simulink model "generic_20240709_1553"  (R2022a)
settings: Solver=ode45  StartTime=0.0  StopTime=inf  RelTol=1e-3  EnableMultiTasking=on
libraries: CarMaker4SL x40, simulink x9, aerolibconvert2 x4, matrix_library x4
(part 1 of 2)
settings Model: Creator=fh  LastModifiedBy=TFTS06
settings SolverCC: AlgebraicLoopSolver=TrustRegion
settings DataIOCC: LimitDataPoints=on  SaveFormat=Array  SignalLoggingSaveFormat=ModelDataLogs  ReturnWorkspaceOutputs=off  SignalLoggingName=sigsOut
settings OptimizationCC: BooleanDataType=off  ExpressionDepthLimit=2147483647  InitFltsAndDblsToZero=on  LifeSpan=inf
settings DebuggingCC: SaveWithParameterizedLinksMsg=none  UnderspecifiedInitializationDetection=Classic  MergeDetectMultiDrivingBlocksExec=none  SignalResolutionControl=TryResolveAllWithWarning  MultiTaskDSMMsg=warning  MultiTaskCondExecSysMsg=none  FcnCallInpInsideContextMsg=warning  UnconnectedInputMsg=warning  UnconnectedOutputMsg=warning  UnconnectedLineMsg=warning  StateNameClashWarn=warning  SFUnexpectedBacktrackingDiag=warning  SFNoUnconditionalDefaultTransitionDiag=warning  SFMachineParentedDataDiag=warning  ArithmeticOperatorsInVariantConditions=warning
settings HardwareCC: ProdBitPerPointer=32  ProdBitPerSizeT=32  ProdBitPerPtrDiffT=32  ProdLargestAtomicFloat=None  ProdIntDivRoundTo=Undefined  ProdEndianess=Unspecified  ProdWordSize=32  ProdHWDeviceType=32-bit Generic  TargetUnknown=on
settings ModelReferenceCC: PropagateSignalLabelsOutOfModel=off
settings SFSimCC: SimUseLocalCustomCode=off  CustomCodeUndefinedFunction=UseInterfaceOnly
settings RTWCC: RTWUseLocalCustomCode=off
settings CodeAppCC: MaxIdLength=63  StateflowObjectComments=on
settings GRTTargetCC: TargetFcnLib=ansi_tfl_tmw.mat  TargetLangStandard=C89/C90 (ANSI)  CombineOutputUpdateFcns=off  GRTInterface=on
settings ConfigComp: CovMetricSettings=dw  CovSaveCumulativeToWorkspaceVar=on  CovSaveSingleToWorkspaceVar=on  CovExternalEMLEnable=off

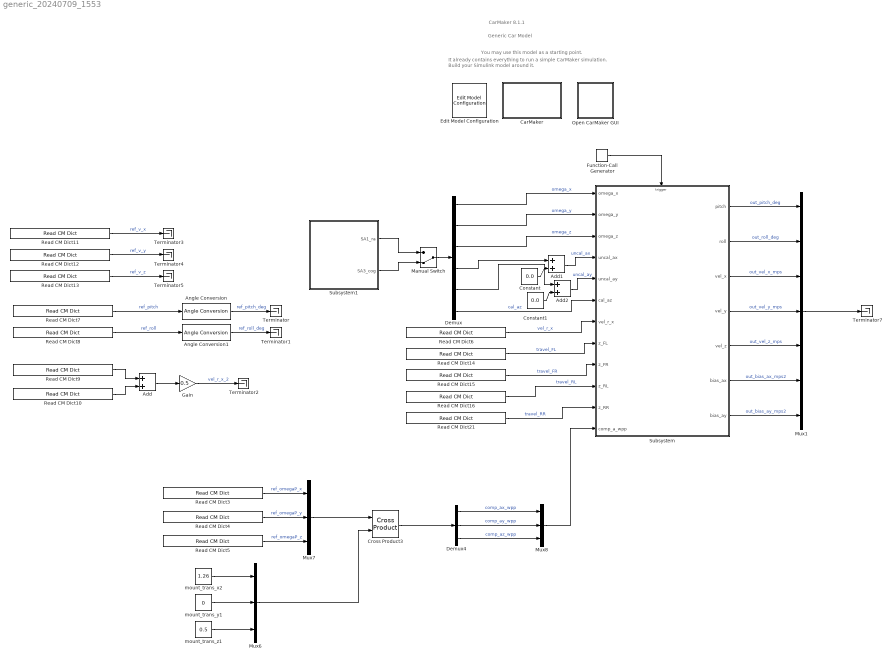
== system generic_20240709_1553 ==
  note: Generic Car Model
  note: You may use this model as a starting point.
  note: It already contains everything to run a simple CarMaker simulation.
      | Build your Simulink model around it.
  note: CarMaker 8.1.1
  Add : Sum
  Add1 : Sum
  Add2 : Sum
  Angle Conversion : aerolibconvert2/Angle Conversion  IU=rad  OU=deg
  Angle Conversion1 : aerolibconvert2/Angle Conversion  IU=rad  OU=deg
  CarMaker : Subsystem  TreatAsAtomicUnit=on
      mask Display: image(imread('CarMakerSys.png'));
  Constant : Constant  Value=0.0
  Constant1 : Constant  Value=0.0
  Cross Product3 : matrix_library/Cross Product
      settings: SourceProductBaseCode=SL
  Demux : Demux  Outputs=6
  Demux4 : Demux  Outputs=3
  Edit Model Configuration : CarMaker4SL/Edit Model Configuration  SFunctionModules=''
  Function-Call Generator : simulink/Ports & Subsystems/Function-Call Generator  sample_time=0.01  numberOfIterations=1  DisallowWideOutput=off
  Gain : Gain  Gain=0.5
  Manual Switch : ManualSwitch  CurrentSetting=0
  Mux1 : Mux  Inputs=7
  Mux6 : Mux  Inputs=3
  Mux7 : Mux  Inputs=3
  Mux8 : Mux  Inputs=3
  Open CarMaker GUI : Subsystem  LoadFcn=if ~length(which('cmself')), cmenv; end
      settings: OpenFcn=cmblockmagic('gui_fix_display'); CM_Simulink
      mask Display: image(imread('CarMakerGUI.png'));
  Read CM Dict10 : CarMaker4SL/Read CM Dict  xname=Car.vRR  xsync=off
  Read CM Dict11 : CarMaker4SL/Read CM Dict  xname=Sensor.Inertial.SA1.Vel_B.x  xsync=off
  Read CM Dict12 : CarMaker4SL/Read CM Dict  xname=Sensor.Inertial.SA1.Vel_B.y  xsync=off
  Read CM Dict13 : CarMaker4SL/Read CM Dict  xname=Sensor.Inertial.SA1.Vel_B.z  xsync=off
  Read CM Dict14 : CarMaker4SL/Read CM Dict  xname=Car.DampFL.l_kin  xsync=off
  Read CM Dict15 : CarMaker4SL/Read CM Dict  xname=Car.DampFR.l_kin  xsync=off
  Read CM Dict16 : CarMaker4SL/Read CM Dict  xname=Car.DampRL.l_kin  xsync=off
  Read CM Dict21 : CarMaker4SL/Read CM Dict  xname=Car.DampRR.l_kin  xsync=off
  Read CM Dict3 : CarMaker4SL/Read CM Dict  xname=Sensor.Inertial.SA1.Alpha_B.x  xsync=off
  Read CM Dict4 : CarMaker4SL/Read CM Dict  xname=Sensor.Inertial.SA1.Alpha_B.y  xsync=off
  Read CM Dict5 : CarMaker4SL/Read CM Dict  xname=Sensor.Inertial.SA1.Alpha_B.z  xsync=off
  Read CM Dict6 : CarMaker4SL/Read CM Dict  xname=Car.vx  xsync=off
  Read CM Dict7 : CarMaker4SL/Read CM Dict  xname=Car.Pitch  xsync=off
  Read CM Dict8 : CarMaker4SL/Read CM Dict  xname=Car.Roll  xsync=off
  Read CM Dict9 : CarMaker4SL/Read CM Dict  xname=Car.vRL  xsync=off
  Subsystem : Subsystem
  Subsystem1 : Subsystem
  Terminator{,1..5,7} (7 alike) : Terminator
  mount_trans_x2 : Constant  Value=1.26
  mount_trans_y1 : Constant  Value=0
  mount_trans_z1 : Constant  Value=0.5
  wires:
  Add1/1 -> Subsystem/4(uncal_ax)  "uncal_ax"
  Add2/1 -> Subsystem/5(uncal_ay)  "uncal_ay"
  Read CM Dict6/1 -> Subsystem/7(vel_r_x)  "vel_r_x"
  Read CM Dict7/1 -> Angle Conversion/1  "ref_pitch"
  Read CM Dict8/1 -> Angle Conversion1/1  "ref_roll"
  Subsystem/1(pitch) -> Mux1/1  "out_pitch_deg"
  Subsystem/7(bias_ay) -> Mux1/7  "out_bias_ay_mps2"
  Subsystem/6(bias_ax) -> Mux1/6  "out_bias_ax_mps2"
  Subsystem/4(vel_y) -> Mux1/4  "out_vel_y_mps"
  Subsystem/3(vel_x) -> Mux1/3  "out_vel_x_mps"
  Mux1/1 -> Terminator7/1
  Subsystem/5(vel_z) -> Mux1/5  "out_vel_z_mps"
  Subsystem/2(roll) -> Mux1/2  "out_roll_deg"
  Function-Call Generator/1 -> Subsystem/Trigger
  Angle Conversion/1 -> Terminator/1  "ref_pitch_deg"
  Angle Conversion1/1 -> Terminator1/1  "ref_roll_deg"
  Read CM Dict9/1 -> Add/1
  Read CM Dict10/1 -> Add/2
  Add/1 -> Gain/1
  Gain/1 -> Terminator2/1  "vel_r_x_2"
  Read CM Dict11/1 -> Terminator3/1  "ref_v_x"
  Read CM Dict13/1 -> Terminator5/1  "ref_v_z"
  Read CM Dict12/1 -> Terminator4/1  "ref_v_y"
  Constant/1 -> Add1/2
  Read CM Dict14/1 -> Subsystem/8(z_FL)  "travel_FL"
  Read CM Dict15/1 -> Subsystem/9(z_FR)  "travel_FR"
  Read CM Dict16/1 -> Subsystem/10(z_RL)  "travel_RL"
  Read CM Dict21/1 -> Subsystem/11(z_RR)  "travel_RR"
  Constant1/1 -> Add2/2
  Demux/1 -> Subsystem/1(omega_x)  "omega_x"
  Demux/2 -> Subsystem/2(omega_y)  "omega_y"
  Demux/3 -> Subsystem/3(omega_z)  "omega_z"
  Demux/4 -> Add1/1
  Demux/5 -> Add2/1
  Demux/6 -> Subsystem/6(cal_az)  "cal_az"
  Manual Switch/1 -> Demux/1
  Subsystem1/1(SA1_ra) -> Manual Switch/1
  Subsystem1/2(SA3_cog) -> Manual Switch/2
  Cross Product3/1 -> Demux4/1
  Read CM Dict5/1 -> Mux7/3  "ref_omegaP_z"
  Read CM Dict3/1 -> Mux7/1  "ref_omegaP_x"
  Mux8/1 -> Subsystem/12(comp_a_wpp)
  Mux7/1 -> Cross Product3/1
  mount_trans_z1/1 -> Mux6/3
  mount_trans_y1/1 -> Mux6/2
  Read CM Dict4/1 -> Mux7/2  "ref_omegaP_y"
  Demux4/3 -> Mux8/3  "comp_az_wpp"
  Demux4/2 -> Mux8/2  "comp_ay_wpp"
  Mux6/1 -> Cross Product3/2
  mount_trans_x2/1 -> Mux6/1
  Demux4/1 -> Mux8/1  "comp_ax_wpp"

== system generic_20240709_1553/CarMaker ==
  CM_FIRST : Subsystem
  CM_LAST : Subsystem
  DrivMan : Subsystem
  Ground : Ground
  IPG Vehicle : Subsystem  TreatAsAtomicUnit=on
  Terminator : Terminator
  VehicleControl : Subsystem
  wires:
  DrivMan/2(DrivMan.Out) -> VehicleControl/2(DrivMan.In)
  DrivMan/1(Sync_Out) -> VehicleControl/1(Sync_In)
  CM_FIRST/2(Env.Misc) -> DrivMan/2(Env.Misc)
  CM_FIRST/1(Sync_Out) -> DrivMan/1(Sync_In)
  CM_LAST/1(Sync_Out) -> Terminator/1
  Ground/1 -> CM_FIRST/1(Sync_In)
  IPG Vehicle/1(Sync_Out) -> CM_LAST/1(Sync_In)
  VehicleControl/1(Sync_Out) -> IPG Vehicle/1(Sync_In)
  VehicleControl/3(VhclCtrl.Steering) -> IPG Vehicle/3(VhclCtrl.Steering)
  VehicleControl/4(Vhcl.Wheel.In) -> IPG Vehicle/4(Vhcl.Wheel.In)
  VehicleControl/5(Vhcl.Misc) -> IPG Vehicle/5(Vhcl.Misc)
  VehicleControl/6(VhclCtrl.Brake) -> IPG Vehicle/6(VhclCtrl.Brake)
  VehicleControl/7(VhclCtrl.PT) -> IPG Vehicle/7(VhclCtrl.PT)
  VehicleControl/2(Vhcl.Model.Source) -> IPG Vehicle/2(Vhcl.Model.Source)

== system generic_20240709_1553/Open CarMaker GUI ==
  S-Function : S-Function  FunctionName=cm_gui  SFunctionDeploymentMode=off  EnableBusSupport=off

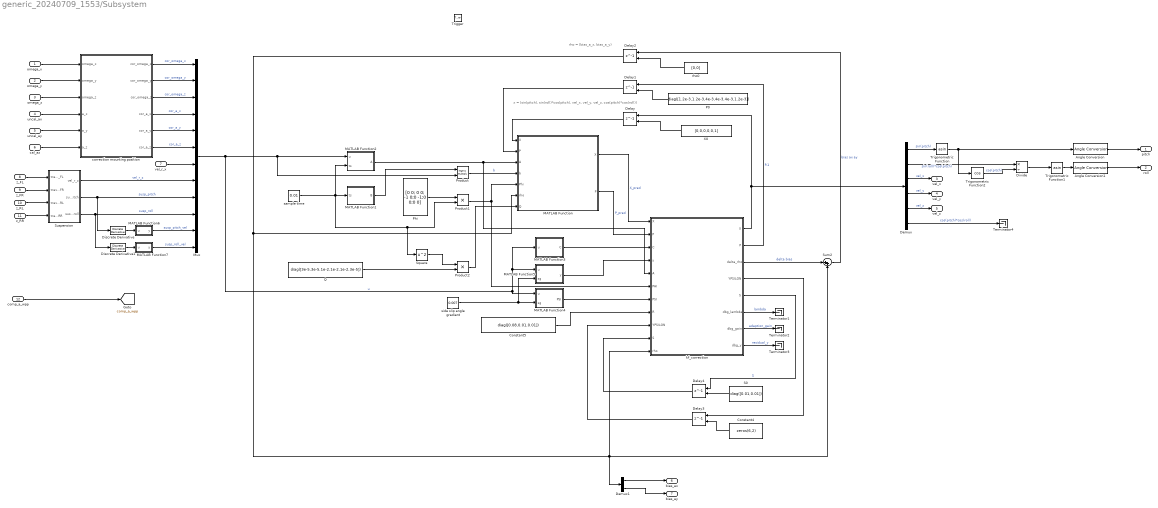
== system generic_20240709_1553/Subsystem ==
  note: rho = (bias_a_x, bias_a_y)
  note: x = (sin(pitch), sin(roll)*cos(pitch), vel_x, vel_y, vel_z, cos(pitch)*cos(roll))
  omega_x : Inport
  omega_y : Inport  Port=2
  omega_z : Inport  Port=3
  uncal_ax : Inport  Port=4
  uncal_ay : Inport  Port=5
  cal_az : Inport  Port=6
  vel_r_x : Inport  Port=7
  z_FL : Inport  Port=8
  z_FR : Inport  Port=9
  z_RL : Inport  Port=10
  z_RR : Inport  Port=11
  comp_a_wpp : Inport  Port=12
  Trigger : TriggerPort  TriggerType=function-call  VariantControl=(inherit)  PortDimensions=1
  Angle Conversion : aerolibconvert2/Angle Conversion  IU=rad  OU=deg
  Angle Conversion1 : aerolibconvert2/Angle Conversion  IU=rad  OU=deg
  Constant4 : Constant  Value=zeros(6,2)
  Constant5 : Constant  Value=diag([0.08,0.01,0.01])
  Delay{,1..4} (5 alike) : Delay  DelayLength=1  InitialConditionSource=Input port  InitialCondition=0
      settings: InputPortMap=u0,p4
  Demux : Demux  Outputs=6
  Demux1 : Demux  Outputs=2
  Discrete Derivative : simulink/Discrete/Discrete Derivative  gainval=1.0  ICPrevScaledInput=0.0  OutMin=[]  OutMax=[]  OutDataType=fixdt(1, 16)  OutScaling=2^-10  DoSatur=off
  Discrete Derivative1 : simulink/Discrete/Discrete Derivative  gainval=1.0  ICPrevScaledInput=0.0  OutMin=[]  OutMax=[]  OutDataType=fixdt(1, 16)  OutScaling=2^-10  DoSatur=off
  Divide : Product  Inputs=*/
  MATLAB Function : MATLAB Function  TreatAsAtomicUnit=on
  MATLAB Function1 : MATLAB Function  TreatAsAtomicUnit=on
  MATLAB Function2 : MATLAB Function  TreatAsAtomicUnit=on
  MATLAB Function3 : MATLAB Function  TreatAsAtomicUnit=on
  MATLAB Function4 : MATLAB Function  TreatAsAtomicUnit=on
  MATLAB Function5 : MATLAB Function  TreatAsAtomicUnit=on
  MATLAB Function6 : MATLAB Function  TreatAsAtomicUnit=on
  MATLAB Function7 : MATLAB Function  TreatAsAtomicUnit=on
  Mux : Mux  Inputs=12
  P0 : Constant  Value=diag([1.2e-3,1.2e-3,4e-3,4e-3,4e-3,1.2e-3])
  Phi : Constant  Value=[0 0; 0 0; -1 0;0 -1;0 0;0 0]
  Product : Product  Multiplication=Matrix(*)
  Product1 : Product
  Product2 : Product
  Q : Constant  Value=diag([3e-5,3e-5,1e-2,1e-2,1e-2,3e-5])
  S0 : Constant  Value=diag([0.01,0.01])
  Square : Math  Operator=square
  Sum2 : Sum  Inputs=|++
  Suspension : Subsystem
  Terminator{1..4} (4 alike) : Terminator
  Trigonometric Function : Trigonometry  Operator=asin
  Trigonometric Function1 : Trigonometry  Operator=asin
  Trigonometric Function2 : Trigonometry  Operator=cos
  X0 : Constant  Value=[0,0,0,0,0,1]
  correction mounting position : Subsystem
  kf_correction : MATLAB Function  TreatAsAtomicUnit=on
  rho0 : Constant  Value=[0,0]
  sample time : Constant  Value=0.01
  side slip angle gradient : Constant  Value=0.007
  pitch : Outport
  roll : Outport  Port=2
  vel_x : Outport  Port=3
  vel_y : Outport  Port=4
  vel_z : Outport  Port=5
  bias_ax : Outport  Port=6
  bias_ay : Outport  Port=7
  tag scope: comp_a_wpp=global
  wires:
  Demux1/2 -> bias_ay/1
  kf_correction/5(S) -> Delay4/1  "S"
  X0/1 -> Delay/2
  kf_correction/7(dbg_gain) -> Terminator2/1  "adaption_gain"
  Demux/1 -> Trigonometric Function/1  "sin(pitch)"
  P0/1 -> Delay1/2
  Demux/3 -> vel_x/1  "vel_x"
  Product/1 -> MATLAB Function/4(b)  "b"
  kf_correction/1(X) -> Demux/1, Delay/1
  Constant4/1 -> Delay3/2
  Demux/4 -> vel_y/1  "vel_y"
  Divide/1 -> Trigonometric Function1/1
  MATLAB Function2/1(A) -> kf_correction/5(A), MATLAB Function/3(A)
  Phi/1 -> Product1/1
  Demux1/1 -> bias_ax/1
  Delay/1 -> MATLAB Function/1("X ")
  MATLAB Function3/1(C) -> kf_correction/3(C)
  kf_correction/2(P) -> Delay1/1  "P-1"
  Suspension/2(susp_pitch) -> Mux/9, Discrete Derivative/1  "susp_pitch"
  Demux/2 -> Divide/1  "sin(roll)*cos(pitch)"
  Delay4/1 -> kf_correction/10("S ")
  Mux/1 -> MATLAB Function2/1(u), Product/2, MATLAB Function4/1(u), MATLAB Function3/1(u), MATLAB Function5/1(u)  "u"
  Suspension/3(susp_roll) -> Mux/10, Discrete Derivative1/1  "susp_roll"
  kf_correction/3(delta_rho) -> Sum2/1  "delta bias"
  Sum2/1 -> Delay2/1  "bias ax ay"
  Trigonometric Function/1 -> Angle Conversion/1, Trigonometric Function2/1
  Constant5/1 -> kf_correction/8(R)
  MATLAB Function4/1(PSI) -> kf_correction/7(PSI)
  Delay3/1 -> kf_correction/9("YPSILON ")
  Suspension/1(vel_r_z) -> Mux/8  "vel_r_z"
  S0/1 -> Delay4/2
  MATLAB Function1/1(B) -> Product/1
  Delay1/1 -> MATLAB Function/2("P ")
  Product1/1 -> MATLAB Function/5(Phi), kf_correction/6(PHI)
  MATLAB Function/2(P) -> kf_correction/2("P ")  "P_pred"
  Trigonometric Function1/1 -> Angle Conversion1/1
  Demux/5 -> vel_z/1  "vel_z"
  rho0/1 -> Delay2/2
  sample time/1 -> MATLAB Function2/2(ts), Product1/2, Square/1, MATLAB Function1/1(ts)
  MATLAB Function/1(X) -> kf_correction/1("X ")  "X_pred"
  Trigonometric Function2/1 -> Divide/2  "cos(pitch)"
  kf_correction/4(YPSILON) -> Delay3/1
  kf_correction/8(dbg_y) -> Terminator3/1  "residual_y"
  Product2/1 -> MATLAB Function/7(Q)
  Delay2/1 -> MATLAB Function/6(rho), Demux1/1, kf_correction/11(rho), Sum2/2
  MATLAB Function5/1(y) -> kf_correction/4(y)
  correction mounting position/4(cor_a_x) -> Mux/4  "cor_a_x"
  kf_correction/6(dbg_lambda) -> Terminator1/1  "lambda"
  correction mounting position/3(cor_omega_z) -> Mux/3  "cor_omega_z"
  correction mounting position/2(cor_omega_y) -> Mux/2  "cor_omega_y"
  correction mounting position/1(cor_omega_x) -> Mux/1  "cor_omega_x"
  Demux/6 -> Terminator4/1  "cos(pitch)*cos(roll)"
  Angle Conversion1/1 -> roll/1
  Angle Conversion/1 -> pitch/1
  Q/1 -> Product2/2
  side slip angle gradient/1 -> MATLAB Function5/2(sg), MATLAB Function4/2(sg)
  z_FL/1 -> Suspension/1(travel_FL)
  z_FR/1 -> Suspension/2(travel_FR)
  z_RL/1 -> Suspension/3(travel_RL)
  z_RR/1 -> Suspension/4(travel_RR)
  MATLAB Function6/1(y) -> Mux/11  "susp_pitch_vel"
  MATLAB Function7/1(y) -> Mux/12  "susp_roll_vel"
  Discrete Derivative/1 -> MATLAB Function6/1(u)
  Discrete Derivative1/1 -> MATLAB Function7/1(u)
  Square/1 -> Product2/1
  correction mounting position/5(cor_a_y) -> Mux/5  "cor_a_y"
  correction mounting position/6(cor_a_z) -> Mux/6  "cor_a_z"
  vel_r_x/1 -> Mux/7
  omega_x/1 -> correction mounting position/1(omega_x)
  omega_y/1 -> correction mounting position/2(omega_y)
  omega_z/1 -> correction mounting position/3(omega_z)
  uncal_ax/1 -> correction mounting position/4(a_x)
  uncal_ay/1 -> correction mounting position/5(a_y)
  cal_az/1 -> correction mounting position/6(a_z)
  comp_a_wpp/1 -> [comp_a_wpp]

== system generic_20240709_1553/Subsystem1 ==
  Mux : Mux  Inputs=6
  Mux1 : Mux  Inputs=6
  Read CM Dict : CarMaker4SL/Read CM Dict  xname=Sensor.Inertial.SA1.Omega_B.x  xsync=off
  Read CM Dict1 : CarMaker4SL/Read CM Dict  xname=Sensor.Inertial.SA1.Omega_B.y  xsync=off
  Read CM Dict10 : CarMaker4SL/Read CM Dict  xname=Sensor.Inertial.SA3.Acc_B.y  xsync=off
  Read CM Dict11 : CarMaker4SL/Read CM Dict  xname=Sensor.Inertial.SA3.Acc_B.z  xsync=off
  Read CM Dict2 : CarMaker4SL/Read CM Dict  xname=Sensor.Inertial.SA1.Omega_B.z  xsync=off
  Read CM Dict3 : CarMaker4SL/Read CM Dict  xname=Sensor.Inertial.SA1.Acc_B.x  xsync=off
  Read CM Dict4 : CarMaker4SL/Read CM Dict  xname=Sensor.Inertial.SA1.Acc_B.y  xsync=off
  Read CM Dict5 : CarMaker4SL/Read CM Dict  xname=Sensor.Inertial.SA1.Acc_B.z  xsync=off
  Read CM Dict6 : CarMaker4SL/Read CM Dict  xname=Sensor.Inertial.SA3.Omega_B.x  xsync=off
  Read CM Dict7 : CarMaker4SL/Read CM Dict  xname=Sensor.Inertial.SA3.Omega_B.y  xsync=off
  Read CM Dict8 : CarMaker4SL/Read CM Dict  xname=Sensor.Inertial.SA3.Omega_B.z  xsync=off
  Read CM Dict9 : CarMaker4SL/Read CM Dict  xname=Sensor.Inertial.SA3.Acc_B.x  xsync=off
  SA1_ra : Outport
  SA3_cog : Outport  Port=2
  wires:
  Read CM Dict2/1 -> Mux/3  "omega_z"
  Read CM Dict1/1 -> Mux/2  "omega_y"
  Read CM Dict/1 -> Mux/1  "omega_x"
  Read CM Dict5/1 -> Mux/6  "cal_az"
  Read CM Dict4/1 -> Mux/5  "uncal_ax"
  Read CM Dict3/1 -> Mux/4  "uncal_ax"
  Mux1/1 -> SA3_cog/1
  Mux/1 -> SA1_ra/1
  Read CM Dict6/1 -> Mux1/1  "omega_x"
  Read CM Dict7/1 -> Mux1/2  "omega_y"
  Read CM Dict8/1 -> Mux1/3  "omega_z"
  Read CM Dict9/1 -> Mux1/4  "uncal_ax"
  Read CM Dict10/1 -> Mux1/5  "uncal_ax"
  Read CM Dict11/1 -> Mux1/6  "cal_az"

== system generic_20240709_1553/CarMaker/CM_FIRST ==
  Sync_In : Inport
  BusCreator1 : BusCreator  Inputs=8
  BusCreator2 : BusCreator  Inputs=6
  Demux1 : Demux  Outputs=14
      settings: DisplayOption=none
  Environment : S-Function  FunctionName=CM_Sfun  Parameters='Environment'  SFunctionDeploymentMode=off  EnableBusSupport=off
  IoIn : S-Function  FunctionName=CM_Sfun  Parameters='IoIn'  SFunctionDeploymentMode=off  EnableBusSupport=off
  Terminator : Terminator
  Sync_Out : Outport
  Env.Misc : Outport  Port=2
  wires:
  BusCreator2/1 -> Terminator/1  "IF Environment (in)"
  BusCreator1/1 -> Env.Misc/1
  Demux1/14 -> BusCreator2/6  "Env sRoad"
  Demux1/13 -> BusCreator2/5  "Env PoI_GCS Elev"
  Demux1/12 -> BusCreator2/4  "Env PoI_GCS Lat"
  Demux1/11 -> BusCreator2/3  "Env PoI_GCS Long"
  Demux1/10 -> BusCreator2/2  "Env Time"
  Demux1/9 -> BusCreator2/1  "Env yDay"
  Demux1/8 -> BusCreator1/8  "Env WindVel_tot z"
  Demux1/7 -> BusCreator1/7  "Env WindVel_tot y"
  Demux1/6 -> BusCreator1/6  "Env WindVel_tot x"
  Demux1/5 -> BusCreator1/5  "Env SolarRadiation"
  Demux1/4 -> BusCreator1/4  "Env AirHumidity"
  Demux1/3 -> BusCreator1/3  "Env AirPressure"
  Demux1/2 -> BusCreator1/2  "Env AirDensity"
  Demux1/1 -> BusCreator1/1  "Env Temperature"
  Environment/2 -> Demux1/1
  Environment/1 -> Sync_Out/1
  IoIn/1 -> Environment/1
  Sync_In/1 -> IoIn/1

== system generic_20240709_1553/CarMaker/CM_LAST ==
  Sync_In : Inport
  CM_User : S-Function  FunctionName=CM_Sfun  Parameters='CM_User'  SFunctionDeploymentMode=off  EnableBusSupport=off
  IoOut : S-Function  FunctionName=CM_Sfun  Parameters='IoOut'  SFunctionDeploymentMode=off  EnableBusSupport=off
  Sync_Out : Outport
  wires:
  IoOut/1 -> Sync_Out/1
  CM_User/1 -> IoOut/1
  Sync_In/1 -> CM_User/1

== system generic_20240709_1553/CarMaker/DrivMan ==
  note: There's rarely a reason to override DrivMan signals.
      | Use the VehicleControl interface for this purpose.
  Sync_In : Inport
  Env.Misc : Inport  Port=2
  BusCreator : BusCreator  Inputs=17
  Demux : Demux  Outputs=17
      settings: DisplayOption=none
  DrivMan : S-Function  FunctionName=CM_Sfun  Parameters='DrivMan'  SFunctionDeploymentMode=off  EnableBusSupport=off
  Sync_Out : Outport
  DrivMan.Out : Outport  Port=2
  wires:
  Demux/17 -> BusCreator/17  "DrivMan Steering Trq"
  Demux/16 -> BusCreator/16  "DrivMan Steering AngAcc"
  Demux/15 -> BusCreator/15  "DrivMan Steering AngVel"
  Demux/14 -> BusCreator/14  "DrivMan Steering Ang"
  Demux/13 -> BusCreator/13  "DrivMan Gas"
  Demux/12 -> BusCreator/12  "DrivMan Clutch"
  Demux/11 -> BusCreator/11  "DrivMan BrakePark"
  Demux/10 -> BusCreator/10  "DrivMan Brake"
  Demux/9 -> BusCreator/9  "DrivMan GearNo"
  Demux/8 -> BusCreator/8  "DrivMan SelectorCtrl"
  Demux/7 -> BusCreator/7  "DrivMan UserSignal4"
  Demux/6 -> BusCreator/6  "DrivMan UserSignal3"
  Demux/5 -> BusCreator/5  "DrivMan UserSignal2"
  Demux/4 -> BusCreator/4  "DrivMan UserSignal1"
  Demux/3 -> BusCreator/3  "DrivMan UserSignal0"
  Demux/2 -> BusCreator/2  "DrivMan Key"
  Demux/1 -> BusCreator/1  "DrivMan SST"
  Env.Misc/1 -> DrivMan/2
  Sync_In/1 -> DrivMan/1
  DrivMan/1 -> Sync_Out/1
  BusCreator/1 -> DrivMan.Out/1
  DrivMan/2 -> Demux/1

== system generic_20240709_1553/CarMaker/IPG Vehicle ==
  Sync_In : Inport
  Vhcl.Model.Source : Inport  Port=2
  VhclCtrl.Steering : Inport  Port=3
  Vhcl.Wheel.In : Inport  Port=4
  Vhcl.Misc : Inport  Port=5
  VhclCtrl.Brake : Inport  Port=6
  VhclCtrl.PT : Inport  Port=7
  Brake : Subsystem
  CarAndTrailer : Subsystem
  PowerTrain : Subsystem
  Stop Simulation : Stop
  VehicleSource_BuiltIn : simulink/Logic and Bit Operations/Compare To Constant  relop=~=  const=1  OutDataTypeStr=boolean  ZeroCross=off
  Sync_Out : Outport
  wires:
  VhclCtrl.PT/1 -> PowerTrain/3(VhclCtrl.PT)
  Brake/1(Sync_Out) -> PowerTrain/1(Sync_In)
  CarAndTrailer/1(Sync_Out) -> Brake/1(Sync_In)
  CarAndTrailer/2(Brake.IF.In) -> Brake/2(Brake.IF.In)
  VhclCtrl.Brake/1 -> Brake/3(VhclCtrl.Brake)
  PowerTrain/1(Sync_Out) -> Sync_Out/1
  Vhcl.Misc/1 -> CarAndTrailer/4(Vhcl.Misc)
  Vhcl.Wheel.In/1 -> CarAndTrailer/3(Vhcl.Wheel.In)
  VhclCtrl.Steering/1 -> CarAndTrailer/2(VhclCtrl.Steering)
  Sync_In/1 -> CarAndTrailer/1(Sync_In)
  Vhcl.Model.Source/1 -> VehicleSource_BuiltIn/1
  VehicleSource_BuiltIn/1 -> Stop Simulation/1
  Brake/2(Vhcl.Wheel.PT) -> PowerTrain/2(Vhcl.Wheel.PT)

== system generic_20240709_1553/CarMaker/VehicleControl ==
  note: <Your model here>
  note: When implementing a vehicle control model,
      | be sure to add '-disablevehiclecontrol' to the command line arguments
      | in the CarMaker Model Configuration block.
      | Otherwise your model will possibly not see the original DrivMan signals
      | on its inputs, but those of a currently activated C-coded vehicle control model instead.
  Sync_In : Inport
  DrivMan.In : Inport  Port=2
  Bus Creator2 : BusCreator  Inputs=2
  CreateBus Vhcl.Misc : Subsystem
  CreateBus Vhcl.Wheel.In : Subsystem
  CreateBus VhclCtrl : Subsystem
  CreateBus VhclCtrl.PT : Subsystem
  CreateBus VhclCtrl.Steering : Subsystem
  Demux2 : Demux  Outputs=2
      settings: DisplayOption=none
  VehicleControl : S-Function  FunctionName=CM_Sfun  Parameters='VehicleControl'  SFunctionDeploymentMode=off  EnableBusSupport=off
  VehicleControlUpd : S-Function  FunctionName=CM_Sfun  Parameters='VehicleControlUpd'  SFunctionDeploymentMode=off  EnableBusSupport=off
  Sync_Out : Outport
  Vhcl.Model.Source : Outport  Port=2
  VhclCtrl.Steering : Outport  Port=3
  Vhcl.Wheel.In : Outport  Port=4
  Vhcl.Misc : Outport  Port=5
  VhclCtrl.Brake : Outport  Port=6
  VhclCtrl.PT : Outport  Port=7
  wires:
  CreateBus VhclCtrl/1(Out) -> VehicleControlUpd/2
  VehicleControl/2 -> CreateBus VhclCtrl/1(In)
  VehicleControlUpd/2 -> Vhcl.Model.Source/1
  VehicleControlUpd/4 -> CreateBus Vhcl.Wheel.In/1(In1)
  VehicleControlUpd/5 -> CreateBus Vhcl.Misc/1(In1)
  VehicleControlUpd/6 -> Demux2/1
  VehicleControlUpd/7 -> CreateBus VhclCtrl.PT/1(In1)
  VehicleControlUpd/3 -> CreateBus VhclCtrl.Steering/1(In1)
  CreateBus Vhcl.Misc/1(Out1) -> Vhcl.Misc/1
  CreateBus Vhcl.Wheel.In/1(Out1) -> Vhcl.Wheel.In/1
  DrivMan.In/1 -> VehicleControl/2
  VehicleControl/1 -> VehicleControlUpd/1
  Sync_In/1 -> VehicleControl/1
  CreateBus VhclCtrl.PT/1(Out1) -> VhclCtrl.PT/1
  Bus Creator2/1 -> VhclCtrl.Brake/1
  CreateBus VhclCtrl.Steering/1(Out1) -> VhclCtrl.Steering/1
  VehicleControlUpd/1 -> Sync_Out/1
  Demux2/2 -> Bus Creator2/2  "VhclCtrl BrakePark"
  Demux2/1 -> Bus Creator2/1  "VhclCtrl Brake"

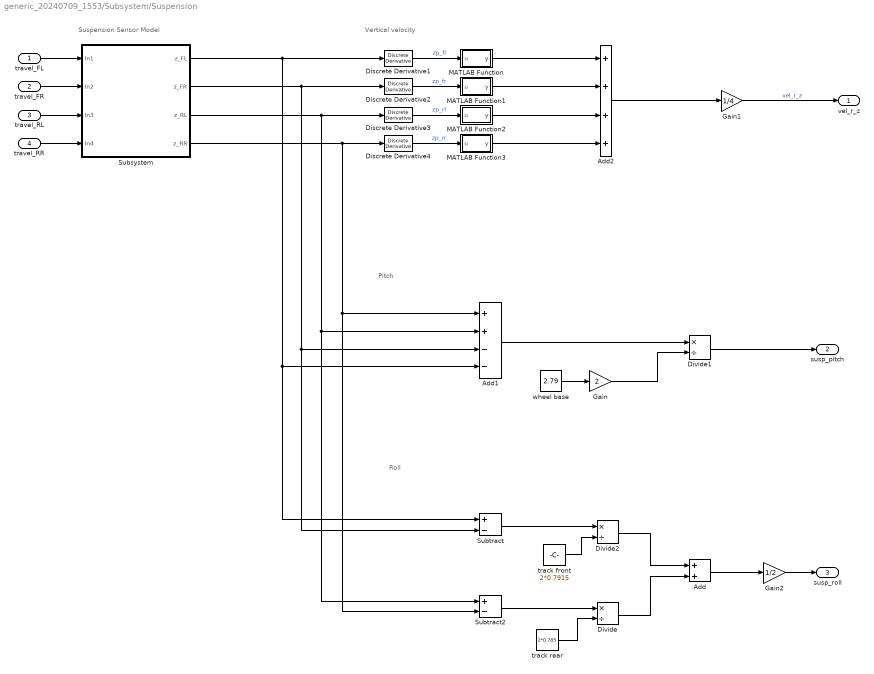
== system generic_20240709_1553/Subsystem/Suspension ==
  note: Vertical velocity
  note: Pitch
  note: Roll
  note: Suspension Sensor Model
  travel_FL : Inport
  travel_FR : Inport  Port=2
  travel_RL : Inport  Port=3
  travel_RR : Inport  Port=4
  Add : Sum
  Add1 : Sum  Inputs=++--
  Add2 : Sum  Inputs=++++
  Discrete Derivative1 : simulink/Discrete/Discrete Derivative  gainval=1.0  ICPrevScaledInput=0.0  OutMin=[-1]  OutMax=[1]  OutDataType=fixdt(1, 16)  OutScaling=2^-10  DoSatur=off
  Discrete Derivative2 : simulink/Discrete/Discrete Derivative  gainval=1.0  ICPrevScaledInput=0.0  OutMin=[]  OutMax=[]  OutDataType=fixdt(1, 16)  OutScaling=2^-10  DoSatur=off
  Discrete Derivative3 : simulink/Discrete/Discrete Derivative  gainval=1.0  ICPrevScaledInput=0.0  OutMin=[]  OutMax=[]  OutDataType=fixdt(1, 16)  OutScaling=2^-10  DoSatur=off
  Discrete Derivative4 : simulink/Discrete/Discrete Derivative  gainval=1.0  ICPrevScaledInput=0.0  OutMin=[]  OutMax=[]  OutDataType=fixdt(1, 16)  OutScaling=2^-10  DoSatur=off
  Divide : Product  Inputs=*/
  Divide1 : Product  Inputs=*/
  Divide2 : Product  Inputs=*/
  Gain : Gain  Gain=2
  Gain1 : Gain  Gain=1/4
  Gain2 : Gain  Gain=1/2
  MATLAB Function : MATLAB Function  TreatAsAtomicUnit=on
  MATLAB Function1 : MATLAB Function  TreatAsAtomicUnit=on
  MATLAB Function2 : MATLAB Function  TreatAsAtomicUnit=on
  MATLAB Function3 : MATLAB Function  TreatAsAtomicUnit=on
  Subsystem : Subsystem
  Subtract : Sum  Inputs=+-
  Subtract2 : Sum  Inputs=+-
  track front : Constant  Value=2*0.7915
  track rear : Constant  Value=2*0.785
  wheel base : Constant  Value=2.79
  vel_r_z : Outport
  susp_pitch : Outport  Port=2
  susp_roll : Outport  Port=3
  wires:
  Add2/1 -> Gain1/1
  Discrete Derivative4/1 -> MATLAB Function3/1(u)  "zp_rr"
  Discrete Derivative3/1 -> MATLAB Function2/1(u)  "zp_rl"
  Discrete Derivative1/1 -> MATLAB Function/1(u)  "zp_fl"
  Gain1/1 -> vel_r_z/1  "vel_r_z"
  Discrete Derivative2/1 -> MATLAB Function1/1(u)  "zp_fr"
  wheel base/1 -> Gain/1
  Gain/1 -> Divide1/2
  Add1/1 -> Divide1/1
  Divide1/1 -> susp_pitch/1
  Subtract/1 -> Divide2/1
  track front/1 -> Divide2/2
  Subtract2/1 -> Divide/1
  track rear/1 -> Divide/2
  Divide2/1 -> Add/1
  Divide/1 -> Add/2
  Gain2/1 -> susp_roll/1
  Add/1 -> Gain2/1
  MATLAB Function/1(y) -> Add2/1
  MATLAB Function1/1(y) -> Add2/2
  MATLAB Function2/1(y) -> Add2/3
  MATLAB Function3/1(y) -> Add2/4
  Subsystem/1(z_FL) -> Subtract/1, Add1/4, Discrete Derivative1/1
  Subsystem/3(z_RL) -> Subtract2/1, Add1/2, Discrete Derivative3/1
  Subsystem/2(z_FR) -> Subtract/2, Add1/3, Discrete Derivative2/1
  Subsystem/4(z_RR) -> Subtract2/2, Add1/1, Discrete Derivative4/1
  travel_FL/1 -> Subsystem/1(In1)
  travel_FR/1 -> Subsystem/2(In2)
  travel_RL/1 -> Subsystem/3(In3)
  travel_RR/1 -> Subsystem/4(In4)

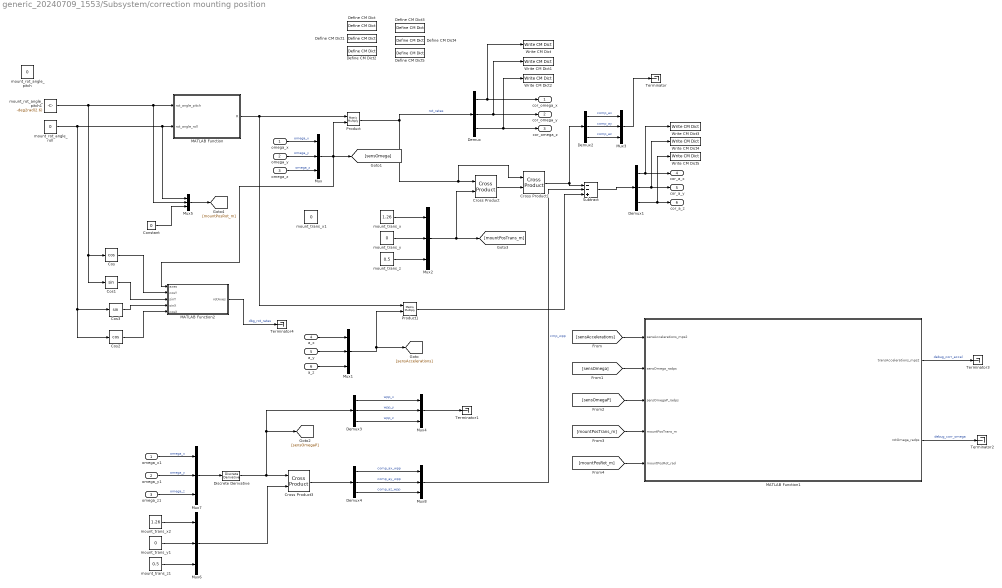
== system generic_20240709_1553/Subsystem/correction mounting position ==
  omega_x : Inport
  omega_y : Inport  Port=2
  omega_z : Inport  Port=3
  a_x : Inport  Port=4
  a_y : Inport  Port=5
  a_z : Inport  Port=6
  Constant : Constant  Value=0
  Cos : Trigonometry  Operator=cos
  Cos1 : Trigonometry
  Cos2 : Trigonometry  Operator=cos
  Cos3 : Trigonometry
  Cross Product : matrix_library/Cross Product
      settings: SourceProductBaseCode=SL
  Cross Product1 : matrix_library/Cross Product
      settings: SourceProductBaseCode=SL
  Cross Product3 : matrix_library/Cross Product
      settings: SourceProductBaseCode=SL
  Define CM Dict : CarMaker4SL/Define CM Dict  xname=MPT_omega_x  xunit=rad/s  xmono=off  xtype=Double4  xdvaplace=None  xnstates=0  xfirststate=0  xinitial=0
  Define CM Dict1 : CarMaker4SL/Define CM Dict  xname=MPT_omega_y  xunit=rad/s  xmono=off  xtype=Double4  xdvaplace=None  xnstates=0  xfirststate=0  xinitial=0
  Define CM Dict2 : CarMaker4SL/Define CM Dict  xname=MPT_omega_z  xunit=rad/s  xmono=off  xtype=Double4  xdvaplace=None  xnstates=0  xfirststate=0  xinitial=0
  Define CM Dict3 : CarMaker4SL/Define CM Dict  xname=MPT_ax  xunit=m/s^2  xmono=off  xtype=Double4  xdvaplace=None  xnstates=0  xfirststate=0  xinitial=0
  Define CM Dict4 : CarMaker4SL/Define CM Dict  xname=MPT_ay  xunit=m/s^2  xmono=off  xtype=Double4  xdvaplace=None  xnstates=0  xfirststate=0  xinitial=0
  Define CM Dict5 : CarMaker4SL/Define CM Dict  xname=MPT_az  xunit=m/s^2  xmono=off  xtype=Double4  xdvaplace=None  xnstates=0  xfirststate=0  xinitial=0
  Demux{,1..4} (5 alike) : Demux  Outputs=3
  Discrete Derivative : simulink/Discrete/Discrete Derivative  gainval=1.0  ICPrevScaledInput=0.0  OutMin=[]  OutMax=[]  OutDataType=fixdt(1, 16)  OutScaling=2^-10  DoSatur=off
  MATLAB Function : MATLAB Function  TreatAsAtomicUnit=on
  MATLAB Function1 : MATLAB Function  TreatAsAtomicUnit=on
  MATLAB Function2 : MATLAB Function  TreatAsAtomicUnit=on
  Mux{,1..8} (9 alike) : Mux  Inputs=3
  Product : Product  Multiplication=Matrix(*)
  Product1 : Product  Multiplication=Matrix(*)
  Subtract : Sum  Inputs=--+
  Terminator{,1..4} (5 alike) : Terminator
  Write CM Dict : CarMaker4SL/Write CM Dict  xname=MPT_omega_x  xsync=off
  Write CM Dict1 : CarMaker4SL/Write CM Dict  xname=MPT_omega_y  xsync=off
  Write CM Dict2 : CarMaker4SL/Write CM Dict  xname=MPT_omega_z  xsync=off
  Write CM Dict3 : CarMaker4SL/Write CM Dict  xname=MPT_ax  xsync=off
  Write CM Dict4 : CarMaker4SL/Write CM Dict  xname=MPT_ay  xsync=off
  Write CM Dict5 : CarMaker4SL/Write CM Dict  xname=MPT_az  xsync=off
  mount_rot_angle_pitch : Constant  Value=0
  mount_rot_angle_pitch1 : Constant  Value=-deg2rad(2.6)
  mount_rot_angle_roll : Constant  Value=0
  mount_trans_x : Constant  Value=1.26
  mount_trans_x1 : Constant  Value=0
  mount_trans_x2 : Constant  Value=1.26
  mount_trans_y : Constant  Value=0
  mount_trans_y1 : Constant  Value=0
  mount_trans_z : Constant  Value=0.5
  mount_trans_z1 : Constant  Value=0.5
  omega_x1 : InportShadow
  omega_y1 : InportShadow  Port=2
  omega_z1 : InportShadow  Port=3
  cor_omega_x : Outport
  cor_omega_y : Outport  Port=2
  cor_omega_z : Outport  Port=3
  cor_a_x : Outport  Port=4
  cor_a_y : Outport  Port=5
  cor_a_z : Outport  Port=6
  wires:
  omega_x/1 -> Mux/1  "omega_x"
  omega_y/1 -> Mux/2  "omega_y"
  omega_z/1 -> Mux/3  "omega_z"
  a_x/1 -> Mux1/1
  a_y/1 -> Mux1/2
  a_z/1 -> Mux1/3
  mount_rot_angle_pitch1/1 -> Cos1/1, Cos/1, Mux5/2, MATLAB Function/1(rot_angle_pitch)
  Mux/1 -> MATLAB Function2/1(axes), [sensOmega], Product/2
  MATLAB Function/1(R) -> Product1/1, Product/1
  Mux1/1 -> [sensAccelerations], Product1/2
  Product/1 -> Demux/1, Cross Product1/1, Cross Product/1  "rot_rates"
  Demux/1 -> Write CM Dict/1, cor_omega_x/1
  Demux/2 -> Write CM Dict1/1, cor_omega_y/1
  Demux/3 -> Write CM Dict2/1, cor_omega_z/1
  mount_trans_x/1 -> Mux2/1
  mount_trans_z/1 -> Mux2/3
  mount_trans_y/1 -> Mux2/2
  Product1/1 -> Subtract/3
  Mux2/1 -> [mountPosTrans_m], Cross Product/2
  Cross Product/1 -> Cross Product1/2
  Cross Product1/1 -> Demux2/1, Subtract/1
  Demux1/3 -> Write CM Dict5/1, cor_a_z/1
  Demux1/2 -> Write CM Dict4/1, cor_a_y/1
  Demux1/1 -> Write CM Dict3/1, cor_a_x/1
  Subtract/1 -> Demux1/1
  Demux2/1 -> Mux3/1  "comp_ax"
  Demux2/2 -> Mux3/2  "comp_ay"
  Demux2/3 -> Mux3/3  "comp_az"
  Mux3/1 -> Terminator/1
  Mux8/1 -> Subtract/2  "cmp_wpp"
  mount_trans_x2/1 -> Mux6/1
  Cross Product3/1 -> Demux4/1
  omega_y1/1 -> Mux7/2  "omega_y"
  Mux7/1 -> Discrete Derivative/1
  omega_x1/1 -> Mux7/1  "omega_x"
  Demux4/3 -> Mux8/3  "comp_az_wpp"
  omega_z1/1 -> Mux7/3  "omega_z"
  Mux6/1 -> Cross Product3/2
  mount_trans_z1/1 -> Mux6/3
  Demux4/2 -> Mux8/2  "comp_ay_wpp"
  mount_trans_y1/1 -> Mux6/2
  Demux4/1 -> Mux8/1  "comp_ax_wpp"
  Demux3/3 -> Mux4/3  "wpp_z"
  Demux3/1 -> Mux4/1  "wpp_x"
  Demux3/2 -> Mux4/2  "wpp_y"
  Discrete Derivative/1 -> [sensOmegaP], Demux3/1, Cross Product3/1
  Mux4/1 -> Terminator1/1
  [sensAccelerations] -> MATLAB Function1/1(sensAccelerations_mps2)
  [sensOmega] -> MATLAB Function1/2(sensOmega_radps)
  [sensOmegaP] -> MATLAB Function1/3(sensOmegaP_radps)
  [mountPosTrans_m] -> MATLAB Function1/4(mountPosTrans_m)
  [mountPosRot_m] -> MATLAB Function1/5(mountPosRot_rad)
  MATLAB Function1/2(rotOmega_radps) -> Terminator2/1  "debug_corr_omega"
  MATLAB Function1/1(transAccelerations_mps2) -> Terminator3/1  "debug_corr_accel"
  Mux5/1 -> [mountPosRot_m]
  Constant/1 -> Mux5/3
  mount_rot_angle_roll/1 -> Cos2/1, Cos3/1, Mux5/1, MATLAB Function/2(rot_angle_roll)
  MATLAB Function2/1(rotAxes) -> Terminator4/1  "dbg_rot_rates"
  Cos/1 -> MATLAB Function2/2(cosY)
  Cos1/1 -> MATLAB Function2/3(sinY)
  Cos2/1 -> MATLAB Function2/5(cosX)
  Cos3/1 -> MATLAB Function2/4(sinX)

== system generic_20240709_1553/CarMaker/IPG Vehicle/Brake ==
  note: When replacing the entire braking system,
      | be sure to disable the IPG brake model by using the brake
      | model 'Model Manager off' in the vehicle GUI.
  note: <Your model here>
  Sync_In : Inport
  Brake.IF.In : Inport  Port=2
  VhclCtrl.Brake : Inport  Port=3
  Brake : S-Function  FunctionName=CM_Sfun  Parameters='Brake'  SFunctionDeploymentMode=off  EnableBusSupport=off
  BrakeUpd : S-Function  FunctionName=CM_Sfun  Parameters='BrakeUpd'  SFunctionDeploymentMode=off  EnableBusSupport=off
  BusCreator1 : BusCreator  Inputs=16
  CreateBus Vhcl.Wheel.PT : Subsystem
  Demux : Demux  Outputs=16
      settings: DisplayOption=none
  Sync_Out : Outport
  Vhcl.Wheel.PT : Outport  Port=2
  wires:
  Demux/16 -> BusCreator1/16  "Brake IF Trq_DriveSrc_trg d3"
  Demux/15 -> BusCreator1/15  "Brake IF Trq_DriveSrc_trg d2"
  Demux/14 -> BusCreator1/14  "Brake IF Trq_DriveSrc_trg d1"
  Demux/13 -> BusCreator1/13  "Brake IF Trq_DriveSrc_trg d0"
  Demux/12 -> BusCreator1/12  "Brake IF Trq_Reg_trg RR"
  Demux/11 -> BusCreator1/11  "Brake IF Trq_Reg_trg RL"
  Demux/10 -> BusCreator1/10  "Brake IF Trq_Reg_trg FR"
  Demux/9 -> BusCreator1/9  "Brake IF Trq_Reg_trg FL"
  Demux/8 -> BusCreator1/8  "Brake IF Trq_PB RR"
  Demux/7 -> BusCreator1/7  "Brake IF Trq_PB RL"
  Demux/6 -> BusCreator1/6  "Brake IF Trq_PB FR"
  Demux/5 -> BusCreator1/5  "Brake IF Trq_PB FL"
  Demux/4 -> BusCreator1/4  "Brake IF Trq_WB RR"
  Demux/3 -> BusCreator1/3  "Brake IF Trq_WB RL"
  Demux/2 -> BusCreator1/2  "Brake IF Trq_WB FR"
  Demux/1 -> BusCreator1/1  "Brake IF Trq_WB FL"
  Brake/2 -> Demux/1
  BusCreator1/1 -> BrakeUpd/2
  BrakeUpd/1 -> Sync_Out/1
  Brake/1 -> BrakeUpd/1  "Sync"
  Brake.IF.In/1 -> Brake/2
  VhclCtrl.Brake/1 -> Brake/3
  Sync_In/1 -> Brake/1
  BrakeUpd/2 -> CreateBus Vhcl.Wheel.PT/1(In)
  CreateBus Vhcl.Wheel.PT/1(Out) -> Vhcl.Wheel.PT/1

== system generic_20240709_1553/CarMaker/IPG Vehicle/CarAndTrailer ==
  Sync_In : Inport
  VhclCtrl.Steering : Inport  Port=2
  Vhcl.Wheel.In : Inport  Port=3
  Vhcl.Misc : Inport  Port=4
  CarAndTrailerUpd : Subsystem
  Forces : Subsystem
  Ground : Ground
  Kinematics : Subsystem
  Kinetics : Subsystem
  Steering : Subsystem
  Terminator : Terminator
  Terminator1 : Terminator
  Trailer : Subsystem
  Sync_Out : Outport
  Brake.IF.In : Outport  Port=2
  wires:
  Trailer/9(Car.Hitch.FrcTrq) -> CarAndTrailerUpd/9(Car.Hitch.FrcTrq)
  Trailer/8(Vhcl.Wheel.RR) -> CarAndTrailerUpd/8(Vhcl.Wheel.RR)
  Trailer/7(Vhcl.Wheel.RL) -> CarAndTrailerUpd/7(Vhcl.Wheel.RL)
  Trailer/6(Vhcl.Wheel.FR) -> CarAndTrailerUpd/6(Vhcl.Wheel.FR)
  Trailer/5(Vhcl.Wheel.FL) -> CarAndTrailerUpd/5(Vhcl.Wheel.FL)
  Trailer/4(Vhcl.PoI) -> CarAndTrailerUpd/4(Vhcl.PoI)
  Trailer/3(Vhcl.Motion) -> CarAndTrailerUpd/3(Vhcl.Motion)
  Trailer/2(Vhcl.Steering) -> CarAndTrailerUpd/2(Vhcl.Steering)
  Trailer/1(Sync_Out) -> CarAndTrailerUpd/1(Sync_In)
  CarAndTrailerUpd/2(Brake.IF.In) -> Brake.IF.In/1
  CarAndTrailerUpd/1(Sync_Out) -> Sync_Out/1
  Vhcl.Misc/1 -> Terminator1/1
  Vhcl.Wheel.In/1 -> Terminator/1
  Kinetics/6(WheelCarrier.Misc) -> Trailer/6(WheelCarrier.Misc)
  Kinetics/5(Car.Trq_T2W) -> Trailer/5(Car.Trq_T2W)
  Steering/2(Steer.IF) -> Kinematics/2(Steer.IF)
  Kinetics/4(Car.Fr1) -> Trailer/4(Car.Fr1)
  Kinetics/3(Car.Hitch) -> Trailer/3(Car.Hitch)
  Kinetics/2(Trailer.Load) -> Trailer/2(Trailer.Load)
  VhclCtrl.Steering/1 -> Steering/2(VhclCtrl.Steering)
  Sync_In/1 -> Steering/1(Sync_In)
  Steering/1(Sync_Out) -> Kinematics/1(Sync_In)
  Kinetics/1(Sync_Out) -> Trailer/1(Sync_In)
  Ground/1 -> CarAndTrailerUpd/10(Vhcl.Fr1A)
  Forces/11(FStabi) -> Kinetics/11(FStabi)
  Forces/10(FDamp) -> Kinetics/10(FDamp)
  Forces/9(FSpring) -> Kinetics/9(FSpring)
  Forces/8(TireRR_Out) -> Kinetics/8(TireRR.Out)
  Forces/7(TireRL_Out) -> Kinetics/7(TireRL.Out)
  Forces/6(TireFR_Out) -> Kinetics/6(TireFR.Out)
  Forces/5(TireFL_Out) -> Kinetics/5(TireFL.Out)
  Forces/4(Car.Load) -> Kinetics/4(Car.Load)
  Forces/2(Car.Virtual) -> Kinetics/2(Car.Virtual)
  Kinematics/6(lSpring) -> Forces/6(lSpring)
  Kinematics/7(vDamp) -> Forces/7(vDamp)
  Forces/3(Car.Aero) -> Kinetics/3(Car.Aero)
  Forces/1(Sync_Out) -> Kinetics/1(Sync_In)
  Kinematics/5(TireRR_In) -> Forces/5(TireRR_In)
  Kinematics/4(TireRL_In) -> Forces/4(TireRL_In)
  Kinematics/3(TireFR_In) -> Forces/3(TireFR_In)
  Kinematics/2(TireFL_In) -> Forces/2(TireFL_In)
  Kinematics/1(Sync_Out) -> Forces/1(Sync_In)
  Kinematics/8(lStabi) -> Forces/8(lStabi)
  Forces/12(FBuf) -> Kinetics/12(FBuf)
  Kinematics/9(lBuf) -> Forces/9(lBuf)

== system generic_20240709_1553/CarMaker/IPG Vehicle/PowerTrain ==
  note: When replacing the entire powertrain,
      | be sure to disable the IPG powertrain model by using the powertrain
      | model 'Model Manager off' in the vehicle GUI.
  note: <Your model here>
  Sync_In : Inport
  Vhcl.Wheel.PT : Inport  Port=2
  VhclCtrl.PT : Inport  Port=3
  BusCreator1 : BusCreator  Inputs=42
  Demux1 : Demux  Outputs=42
      settings: DisplayOption=none
  PowerTrain : S-Function  FunctionName=CM_Sfun  Parameters='PowerTrain'  SFunctionDeploymentMode=off  EnableBusSupport=off
  PowerTrainUpd : S-Function  FunctionName=CM_Sfun  Parameters='PowerTrainUpd'  SFunctionDeploymentMode=off  EnableBusSupport=off
  Sync_Out : Outport
  wires:
  BusCreator1/1 -> PowerTrainUpd/2
  Demux1/42 -> BusCreator1/42  "PT IF WRR Trq_BrakeReg_max"
  Demux1/41 -> BusCreator1/41  "PT IF WRR Trq_BrakeReg"
  Demux1/40 -> BusCreator1/40  "PT IF WRR Trq_Supp2WC"
  Demux1/39 -> BusCreator1/39  "PT IF WRR Trq_Drive"
  Demux1/38 -> BusCreator1/38  "PT IF WRR Trq_B2W"
  Demux1/37 -> BusCreator1/37  "PT IF WRR rotv"
  Demux1/36 -> BusCreator1/36  "PT IF WRR rot"
  Demux1/35 -> BusCreator1/35  "PT IF WRL Trq_BrakeReg_max"
  Demux1/34 -> BusCreator1/34  "PT IF WRL Trq_BrakeReg"
  Demux1/33 -> BusCreator1/33  "PT IF WRL Trq_Supp2WC"
  Demux1/32 -> BusCreator1/32  "PT IF WRL Trq_Drive"
  Demux1/31 -> BusCreator1/31  "PT IF WRL Trq_B2W"
  Demux1/30 -> BusCreator1/30  "PT IF WRL rotv"
  Demux1/29 -> BusCreator1/29  "PT IF WRL rot"
  Demux1/28 -> BusCreator1/28  "PT IF WFR Trq_BrakeReg_max"
  Demux1/27 -> BusCreator1/27  "PT IF WFR Trq_BrakeReg"
  Demux1/26 -> BusCreator1/26  "PT IF WFR Trq_Supp2WC"
  Demux1/25 -> BusCreator1/25  "PT IF WFR Trq_Drive"
  Demux1/24 -> BusCreator1/24  "PT IF WFR Trq_B2W"
  Demux1/23 -> BusCreator1/23  "PT IF WFR rotv"
  Demux1/22 -> BusCreator1/22  "PT IF WFR rot"
  Demux1/21 -> BusCreator1/21  "PT IF WFL Trq_BrakeReg_max"
  Demux1/20 -> BusCreator1/20  "PT IF WFL Trq_BrakeReg"
  Demux1/19 -> BusCreator1/19  "PT IF WFL Trq_Supp2WC"
  Demux1/18 -> BusCreator1/18  "PT IF WFL Trq_Drive"
  Demux1/17 -> BusCreator1/17  "PT IF WFL Trq_B2W"
  Demux1/16 -> BusCreator1/16  "PT IF WFL rotv"
  Demux1/15 -> BusCreator1/15  "PT IF WFL rot"
  Demux1/14 -> BusCreator1/14  "PT IF DL_iDiff_mean"
  Demux1/13 -> BusCreator1/13  "PT IF Trq_Supp2BdyEng y"
  Demux1/12 -> BusCreator1/12  "PT IF Trq_Supp2BdyEng x"
  Demux1/11 -> BusCreator1/11  "PT IF Trq_Supp2Bdy1B z"
  Demux1/10 -> BusCreator1/10  "PT IF Trq_Supp2Bdy1B y"
  Demux1/9 -> BusCreator1/9  "PT IF Trq_Supp2Bdy1B x"
  Demux1/8 -> BusCreator1/8  "PT IF Trq_Supp2Bdy1 z"
  Demux1/7 -> BusCreator1/7  "PT IF Trq_Supp2Bdy1 y"
  Demux1/6 -> BusCreator1/6  "PT IF Trq_Supp2Bdy1 x"
  Demux1/5 -> BusCreator1/5  "PT IF Engine_rotv"
  Demux1/4 -> BusCreator1/4  "PT IF GearNo"
  Demux1/3 -> BusCreator1/3  "PT IF OperationError"
  Demux1/2 -> BusCreator1/2  "PT IF OperationState"
  Demux1/1 -> BusCreator1/1  "PT IF Ignition"
  Sync_In/1 -> PowerTrain/1
  PowerTrain/2 -> Demux1/1
  PowerTrainUpd/1 -> Sync_Out/1
  PowerTrain/1 -> PowerTrainUpd/1  "Sync"
  VhclCtrl.PT/1 -> PowerTrain/3
  Vhcl.Wheel.PT/1 -> PowerTrain/2

== system generic_20240709_1553/CarMaker/VehicleControl/CreateBus Vhcl.Misc ==
  In1 : Inport
  BusCreator : BusCreator  Inputs=11
  Demux : Demux  Outputs=11
      settings: DisplayOption=none
  Out1 : Outport
  wires:
  Demux/11 -> BusCreator/11  "Vhcl Wind_vel_0 z"
  Demux/10 -> BusCreator/10  "Vhcl Wind_vel_0 y"
  Demux/9 -> BusCreator/9  "Vhcl Wind_vel_0 x"
  Demux/8 -> BusCreator/8  "Vhcl Trq_DL2BdyEng y"
  Demux/7 -> BusCreator/7  "Vhcl Trq_DL2BdyEng x"
  Demux/6 -> BusCreator/6  "Vhcl Trq_DL2Bdy1B z"
  Demux/5 -> BusCreator/5  "Vhcl Trq_DL2Bdy1B y"
  Demux/4 -> BusCreator/4  "Vhcl Trq_DL2Bdy1B x"
  Demux/3 -> BusCreator/3  "Vhcl Trq_DL2Bdy1 z"
  Demux/2 -> BusCreator/2  "Vhcl Trq_DL2Bdy1 y"
  Demux/1 -> BusCreator/1  "Vhcl Trq_DL2Bdy1 x"
  In1/1 -> Demux/1
  BusCreator/1 -> Out1/1

== system generic_20240709_1553/CarMaker/VehicleControl/CreateBus Vhcl.Wheel.In ==
  In1 : Inport
  Bus Creator1 : BusCreator  Inputs=12
  Demux1 : Demux  Outputs=12
      settings: DisplayOption=none
  Out1 : Outport
  wires:
  Demux1/12 -> Bus Creator1/12  "Vhcl Wheel RR rotv"
  Demux1/11 -> Bus Creator1/11  "Vhcl Wheel RR Trq_DL2WC"
  Demux1/10 -> Bus Creator1/10  "Vhcl Wheel RR Trq_B2WC"
  Demux1/9 -> Bus Creator1/9  "Vhcl Wheel RL rotv"
  Demux1/8 -> Bus Creator1/8  "Vhcl Wheel RL Trq_DL2WC"
  Demux1/7 -> Bus Creator1/7  "Vhcl Wheel RL Trq_B2WC"
  Demux1/6 -> Bus Creator1/6  "Vhcl Wheel FR rotv"
  Demux1/5 -> Bus Creator1/5  "Vhcl Wheel FR Trq_DL2WC"
  Demux1/4 -> Bus Creator1/4  "Vhcl Wheel FR Trq_B2WC"
  Demux1/3 -> Bus Creator1/3  "Vhcl Wheel FL rotv"
  In1/1 -> Demux1/1
  Bus Creator1/1 -> Out1/1
  Demux1/2 -> Bus Creator1/2  "Vhcl Wheel FL Trq_DL2WC"
  Demux1/1 -> Bus Creator1/1  "Vhcl Wheel FL Trq_B2WC"

== system generic_20240709_1553/CarMaker/VehicleControl/CreateBus VhclCtrl ==
  In : Inport
  BusCreator : BusCreator  Inputs=29
  Demux : Demux  Outputs=29
      settings: DisplayOption=none
  Out : Outport
  wires:
  In/1 -> Demux/1
  BusCreator/1 -> Out/1
  Demux/1 -> BusCreator/1  "VhclCtrl SST"
  Demux/2 -> BusCreator/2  "VhclCtrl Key"
  Demux/3 -> BusCreator/3  "VhclCtrl UserSignal0"
  Demux/4 -> BusCreator/4  "VhclCtrl UserSignal1"
  Demux/5 -> BusCreator/5  "VhclCtrl UserSignal2"
  Demux/6 -> BusCreator/6  "VhclCtrl UserSignal3"
  Demux/7 -> BusCreator/7  "VhclCtrl UserSignal4"
  Demux/8 -> BusCreator/8  "VhclCtrl GearNo"
  Demux/9 -> BusCreator/9  "VhclCtrl SelectorCtrl"
  Demux/10 -> BusCreator/10  "VhclCtrl Brake"
  Demux/11 -> BusCreator/11  "VhclCtrl BrakePark"
  Demux/12 -> BusCreator/12  "VhclCtrl Clutch"
  Demux/13 -> BusCreator/13  "VhclCtrl Gas"
  Demux/14 -> BusCreator/14  "VhclCtrl Steering Ang"
  Demux/15 -> BusCreator/15  "VhclCtrl Steering AngVel"
  Demux/16 -> BusCreator/16  "VhclCtrl Steering AngAcc"
  Demux/17 -> BusCreator/17  "VhclCtrl Steering Trq"
  Demux/18 -> BusCreator/18  "VhclCtrl Lights LowBeam"
  Demux/19 -> BusCreator/19  "VhclCtrl Lights HighBeam"
  Demux/20 -> BusCreator/20  "VhclCtrl Lights Daytime"
  Demux/21 -> BusCreator/21  "VhclCtrl Lights ParkL"
  Demux/22 -> BusCreator/22  "VhclCtrl Lights ParkR"
  Demux/23 -> BusCreator/23  "VhclCtrl Lights IndL"
  Demux/24 -> BusCreator/24  "VhclCtrl Lights IndR"
  Demux/25 -> BusCreator/25  "VhclCtrl Lights FogFrontL"
  Demux/26 -> BusCreator/26  "VhclCtrl Lights FogFrontR"
  Demux/27 -> BusCreator/27  "VhclCtrl Lights FogRear"
  Demux/28 -> BusCreator/28  "VhclCtrl Lights Brake"
  Demux/29 -> BusCreator/29  "VhclCtrl Lights Reverse"

== system generic_20240709_1553/CarMaker/VehicleControl/CreateBus VhclCtrl.PT ==
  In1 : Inport
  BusCreator1 : BusCreator  Inputs=12
  Demux1 : Demux  Outputs=12
      settings: DisplayOption=none
  Out1 : Outport
  wires:
  Demux1/12 -> BusCreator1/12  "VhclCtrl Brake"
  Demux1/11 -> BusCreator1/11  "VhclCtrl Gas"
  Demux1/10 -> BusCreator1/10  "VhclCtrl Clutch"
  Demux1/9 -> BusCreator1/9  "VhclCtrl SelectorCtrl"
  Demux1/8 -> BusCreator1/8  "VhclCtrl GearNo"
  Demux1/7 -> BusCreator1/7  "VhclCtrl UserSignal4"
  Demux1/6 -> BusCreator1/6  "VhclCtrl UserSignal3"
  Demux1/5 -> BusCreator1/5  "VhclCtrl UserSignal2"
  Demux1/4 -> BusCreator1/4  "VhclCtrl UserSignal1"
  Demux1/3 -> BusCreator1/3  "VhclCtrl UserSignal0"
  Demux1/2 -> BusCreator1/2  "VhclCtrl Key"
  Demux1/1 -> BusCreator1/1  "VhclCtrl SST"
  In1/1 -> Demux1/1
  BusCreator1/1 -> Out1/1

== system generic_20240709_1553/CarMaker/VehicleControl/CreateBus VhclCtrl.Steering ==
  In1 : Inport
  Bus Creator : BusCreator  Inputs=5
  Demux : Demux  Outputs=5
      settings: DisplayOption=none
  Out1 : Outport
  wires:
  In1/1 -> Demux/1
  Bus Creator/1 -> Out1/1
  Demux/1 -> Bus Creator/1  "VhclCtrl Steering Ang"
  Demux/5 -> Bus Creator/5  "VhclCtrl Steering SteerByTrq"
  Demux/3 -> Bus Creator/3  "VhclCtrl Steering AngAcc"
  Demux/2 -> Bus Creator/2  "VhclCtrl Steering AngVel"
  Demux/4 -> Bus Creator/4  "VhclCtrl Steering Trq"

== system generic_20240709_1553/Subsystem/Suspension/Subsystem ==
  In1 : Inport
  In2 : Inport  Port=2
  In3 : Inport  Port=3
  In4 : Inport  Port=4
  Add3 : Sum
  Add4 : Sum
  Demux : Demux
  Mux{,1..3} (4 alike) : Mux
  Product : Product
  gradSuspFront_mpm : Constant  Value=1.1853
  gradSuspRear_mpm : Constant  Value=1.05334962160862
  offSuspFront_m : Constant  Value=0.3061
  offSuspRear_m : Constant  Value=0.362
  offZeroLoadFront_m : Constant  Value=-0.689
  offZeroLoadRear_m : Constant  Value=-0.689
  z_FL : Outport
  z_FR : Outport  Port=2
  z_RL : Outport  Port=3
  z_RR : Outport  Port=4
  wires:
  offZeroLoadRear_m/1 -> Mux/4, Mux/3
  Demux/2 -> z_FR/1  "z_FR"
  Demux/4 -> z_RR/1  "z_RR"
  Mux/1 -> Add4/2
  offSuspFront_m/1 -> Mux1/1, Mux1/2
  In1/1 -> Mux3/1
  Mux1/1 -> Add3/2
  gradSuspFront_mpm/1 -> Mux2/1, Mux2/2
  offSuspRear_m/1 -> Mux1/4, Mux1/3
  gradSuspRear_mpm/1 -> Mux2/4, Mux2/3
  Product/1 -> Add3/1
  offZeroLoadFront_m/1 -> Mux/1, Mux/2
  Add3/1 -> Add4/1
  Add4/1 -> Demux/1
  Mux3/1 -> Product/1
  Demux/1 -> z_FL/1  "z_FL"
  Mux2/1 -> Product/2
  In3/1 -> Mux3/3
  In2/1 -> Mux3/2
  Demux/3 -> z_RL/1  "z_RL"
  In4/1 -> Mux3/4

== system generic_20240709_1553/CarMaker/IPG Vehicle/Brake/CreateBus Vhcl.Wheel.PT ==
  In : Inport
  BusCreator1 : BusCreator  Inputs=20
  Demux1 : Demux  Outputs=20
      settings: DisplayOption=none
  Out : Outport
  wires:
  Demux1/20 -> BusCreator1/20  "Vhcl Trq_DriveSrc_trg d3"
  Demux1/19 -> BusCreator1/19  "Vhcl Trq_DriveSrc_trg d2"
  Demux1/18 -> BusCreator1/18  "Vhcl Trq_DriveSrc_trg d1"
  Demux1/17 -> BusCreator1/17  "Vhcl Trq_DriveSrc_trg d0"
  Demux1/16 -> BusCreator1/16  "Vhcl Wheel RR WhlBearing"
  Demux1/15 -> BusCreator1/15  "Vhcl Wheel RR Trq_T2W"
  Demux1/14 -> BusCreator1/14  "Vhcl Wheel RR Trq_BrakeReg_trg"
  Demux1/13 -> BusCreator1/13  "Vhcl Wheel RR Trq_Brake"
  Demux1/12 -> BusCreator1/12  "Vhcl Wheel RL WhlBearing"
  Demux1/11 -> BusCreator1/11  "Vhcl Wheel RL Trq_T2W"
  Demux1/10 -> BusCreator1/10  "Vhcl Wheel RL Trq_BrakeReg_trg"
  Demux1/9 -> BusCreator1/9  "Vhcl Wheel RL Trq_Brake"
  Demux1/8 -> BusCreator1/8  "Vhcl Wheel FR WhlBearing"
  Demux1/7 -> BusCreator1/7  "Vhcl Wheel FR Trq_T2W"
  Demux1/6 -> BusCreator1/6  "Vhcl Wheel FR Trq_BrakeReg_trg"
  Demux1/5 -> BusCreator1/5  "Vhcl Wheel FR Trq_Brake"
  Demux1/4 -> BusCreator1/4  "Vhcl Wheel FL WhlBearing"
  Demux1/3 -> BusCreator1/3  "Vhcl Wheel FL Trq_T2W"
  Demux1/2 -> BusCreator1/2  "Vhcl Wheel FL Trq_BrakeReg_trg"
  Demux1/1 -> BusCreator1/1  "Vhcl Wheel FL Trq_Brake"
  BusCreator1/1 -> Out/1
  In/1 -> Demux1/1

== system generic_20240709_1553/CarMaker/IPG Vehicle/CarAndTrailer/CarAndTrailerUpd ==
  Sync_In : Inport
  Vhcl.Steering : Inport  Port=2
  Vhcl.Motion : Inport  Port=3
  Vhcl.PoI : Inport  Port=4
  Vhcl.Wheel.FL : Inport  Port=5
  Vhcl.Wheel.FR : Inport  Port=6
  Vhcl.Wheel.RL : Inport  Port=7
  Vhcl.Wheel.RR : Inport  Port=8
  Car.Hitch.FrcTrq : Inport  Port=9
  Vhcl.Fr1A : Inport  Port=10
  CarAndTrailerUpd : S-Function  FunctionName=CM_Sfun  Parameters='CarAndTrUpd'  SFunctionDeploymentMode=off  EnableBusSupport=off
  CreateBus Brake.IF.In : Subsystem
  Sync_Out : Outport
  Brake.IF.In : Outport  Port=2
  wires:
  Vhcl.Fr1A/1 -> CarAndTrailerUpd/10  "user vehicle only"
  Vhcl.Steering/1 -> CarAndTrailerUpd/2
  Vhcl.Motion/1 -> CarAndTrailerUpd/3
  Vhcl.PoI/1 -> CarAndTrailerUpd/4
  Vhcl.Wheel.FL/1 -> CarAndTrailerUpd/5
  Vhcl.Wheel.FR/1 -> CarAndTrailerUpd/6
  Car.Hitch.FrcTrq/1 -> CarAndTrailerUpd/9
  Vhcl.Wheel.RR/1 -> CarAndTrailerUpd/8
  Vhcl.Wheel.RL/1 -> CarAndTrailerUpd/7
  CarAndTrailerUpd/2 -> CreateBus Brake.IF.In/1(In)
  CreateBus Brake.IF.In/1(Out) -> Brake.IF.In/1
  CarAndTrailerUpd/1 -> Sync_Out/1
  Sync_In/1 -> CarAndTrailerUpd/1

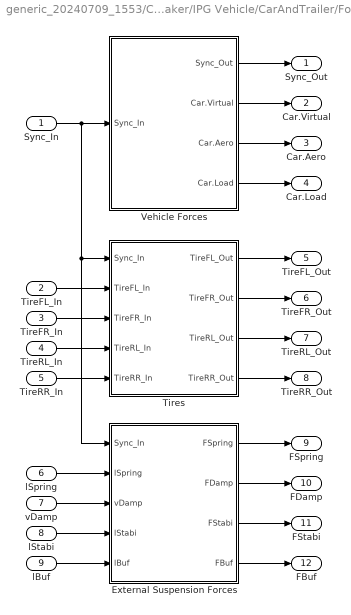
== system generic_20240709_1553/CarMaker/IPG Vehicle/CarAndTrailer/Forces ==
  Sync_In : Inport
  TireFL_In : Inport  Port=2
  TireFR_In : Inport  Port=3
  TireRL_In : Inport  Port=4
  TireRR_In : Inport  Port=5
  lSpring : Inport  Port=6
  vDamp : Inport  Port=7
  lStabi : Inport  Port=8
  lBuf : Inport  Port=9
  External Suspension Forces : Subsystem
  Tires : Subsystem
  Vehicle Forces : Subsystem
  Sync_Out : Outport
  Car.Virtual : Outport  Port=2
  Car.Aero : Outport  Port=3
  Car.Load : Outport  Port=4
  TireFL_Out : Outport  Port=5
  TireFR_Out : Outport  Port=6
  TireRL_Out : Outport  Port=7
  TireRR_Out : Outport  Port=8
  FSpring : Outport  Port=9
  FDamp : Outport  Port=10
  FStabi : Outport  Port=11
  FBuf : Outport  Port=12
  wires:
  lBuf/1 -> External Suspension Forces/5(lBuf)
  lStabi/1 -> External Suspension Forces/4(lStabi)
  vDamp/1 -> External Suspension Forces/3(vDamp)
  Tires/4(TireRR_Out) -> TireRR_Out/1
  Tires/3(TireRL_Out) -> TireRL_Out/1
  Tires/2(TireFR_Out) -> TireFR_Out/1
  Tires/1(TireFL_Out) -> TireFL_Out/1
  TireRR_In/1 -> Tires/5(TireRR_In)
  TireRL_In/1 -> Tires/4(TireRL_In)
  TireFR_In/1 -> Tires/3(TireFR_In)
  TireFL_In/1 -> Tires/2(TireFL_In)
  External Suspension Forces/4(FBuf) -> FBuf/1
  Sync_In/1 -> External Suspension Forces/1(Sync_In), Tires/1(Sync_In), Vehicle Forces/1(Sync_In)
  Vehicle Forces/1(Sync_Out) -> Sync_Out/1
  Vehicle Forces/2(Car.Virtual) -> Car.Virtual/1
  Vehicle Forces/3(Car.Aero) -> Car.Aero/1
  Vehicle Forces/4(Car.Load) -> Car.Load/1
  lSpring/1 -> External Suspension Forces/2(lSpring)
  External Suspension Forces/2(FDamp) -> FDamp/1
  External Suspension Forces/3(FStabi) -> FStabi/1
  External Suspension Forces/1(FSpring) -> FSpring/1
